simulink model "SIM_4_TANK"  (R2023b)
settings: Solver=VariableStepAuto  StartTime=0.0  StopTime=1200  RelTol=1e-3
values from neighbouring files (symbols this model uses):
  Ts = 3    [NMPC_FOUR_TANKS.m]
  u0 = [55;75]    [NMPC_FOUR_TANKS.m]
libraries: sharedTrackingLibrary x1, mpclib x1, simulink x1
settings Model: Creator=DELL  LastModifiedBy=akeebismail

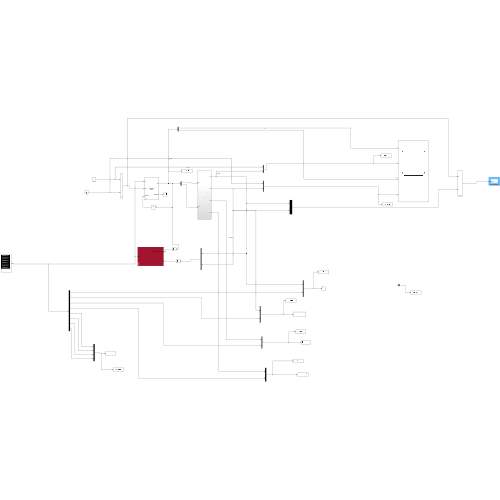
[thumbnail: Simulink's stored preview of the top-level diagram]
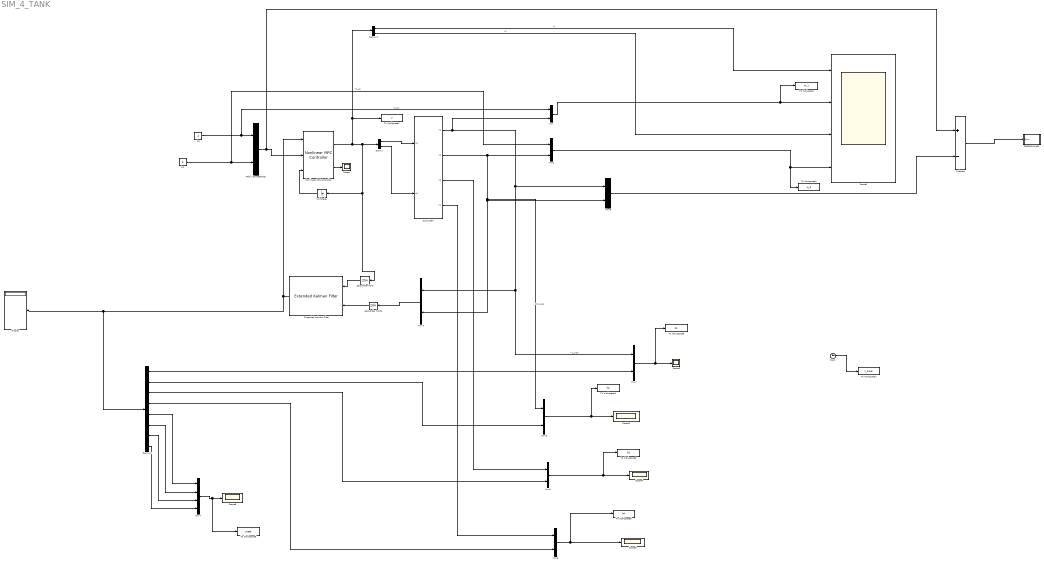
== system SIM_4_TANK ==
  Clock : Clock
  Demux : Demux  Outputs=2
  Demux1 : Demux  Outputs=2
  Demux2 : Demux  Outputs=8
  Display : Display
  Extended Kalman Filter : sharedTrackingLibrary/Extended Kalman Filter  StateTransitionFcn=four_tankStateFcnDT  HasStateTransitionJacobianFcn=off  HasAdditiveProcessNoise=Additive  ProcessNoise=[1e-7;1e-7;1e-7;1e-7;1e-7;1e-7;1e-7;1e-7]  HasTimeVaryingProcessNoise=off  HasStateTransitionFcnExtraArgument=1  InitialState=h0  InitialStateCovariance=[1;1;1;1;1;1;1;1]  MeasurementFcn1=four_tankMeasFcn  HasMeasurementJacobianFcn1=off  HasMeasurementEnablePort1=off  HasAdditiveMeasurementNoise1=Additive  MeasurementNoise1=[1e-2; 1e-2]  HasTimeVaryingMeasurementNoise1=off  HasMeasurementFcnExtraArgument1=0  HasMeasurementWrapping1=off  MeasurementFcn2=myMeasurementFcn  HasMeasurementJacobianFcn2=off  HasMeasurementEnablePort2=off  HasAdditiveMeasurementNoise2=Additive  MeasurementNoise2=1  HasTimeVaryingMeasurementNoise2=off  HasMeasurementFcnExtraArgument2=0  HasMeasurementWrapping2=off  MeasurementFcn3=myMeasurementFcn  HasMeasurementJacobianFcn3=off  HasMeasurementEnablePort3=off  HasAdditiveMeasurementNoise3=Additive  MeasurementNoise3=1  HasTimeVaryingMeasurementNoise3=off  HasMeasurementFcnExtraArgument3=0  HasMeasurementWrapping3=off  MeasurementFcn4=myMeasurementFcn  HasMeasurementJacobianFcn4=off  HasMeasurementEnablePort4=off  HasAdditiveMeasurementNoise4=Additive  MeasurementNoise4=1  HasTimeVaryingMeasurementNoise4=off  HasMeasurementFcnExtraArgument4=0  HasMeasurementWrapping4=off  MeasurementFcn5=myMeasurementFcn  HasMeasurementJacobianFcn5=off  HasMeasurementEnablePort5=off  HasAdditiveMeasurementNoise5=Additive  MeasurementNoise5=1  HasTimeVaryingMeasurementNoise5=off  HasMeasurementFcnExtraArgument5=0  HasMeasurementWrapping5=off  EnableMultirate=off  StateTransitionFcnSampleTime=1  MeasurementFcn1SampleTime=1  MeasurementFcn2SampleTime=1  MeasurementFcn3SampleTime=1  MeasurementFcn4SampleTime=1  MeasurementFcn5SampleTime=1  UseCurrentEstimator=on  OutputStateCovariance=off  DataType=double  SampleTime=Ts  NumberOfMeasurements=1
  Matrix Concatenate : Concatenate  Mode=Multidimensional array  ConcatenateDimension=2
  Mux{,1..6,8} (8 alike) : Mux  Inputs=2
  Mux7 : Mux
  Nonlinear MPC Controller : mpclib/Nonlinear MPC Controller  nlmpcobj=nlobj  UseObjectTs=on  UseMEX=off  md_enabled=off  mvtarget_enabled=off  param_enabled=off  cost_enabled=off  mvseq_enabled=off  stateseq_enabled=off  ovseq_enabled=off  slack_enabled=off  status_enabled=on  ov_min=off  ov_max=off  mv_min=off  mv_max=off  mvrate_min=off  mvrate_max=off  state_min=off  state_max=off  ov_weight=off  mv_weight=off  mvrate_weight=off  ecr_weight=off  nlp_initialize=off
  PERFORMANCE : Subsystem
  Scope{,2..6} (6 alike) : Scope
  Scope1 : Scope  NumInputPorts=4
  Subsystem : Subsystem
  Subtract : Sum  Inputs=+-
  To Workspace : ToWorkspace  VariableName=H_1  SaveFormat=Timeseries  SampleTime=Ts
  To Workspace1 : ToWorkspace  VariableName=H_2  SaveFormat=Timeseries  SampleTime=Ts
  To Workspace2 : ToWorkspace  VariableName=V  SaveFormat=Timeseries  SampleTime=Ts
  To Workspace3 : ToWorkspace  VariableName=h1  SaveFormat=Timeseries  SampleTime=Ts
  To Workspace4 : ToWorkspace  VariableName=h2  SaveFormat=Timeseries  SampleTime=Ts
  To Workspace5 : ToWorkspace  VariableName=h3  SaveFormat=Timeseries  SampleTime=Ts
  To Workspace6 : ToWorkspace  VariableName=h4  SaveFormat=Timeseries  SampleTime=Ts
  To Workspace7 : ToWorkspace  VariableName=t_save  SaveFormat=Timeseries  SampleTime=Ts
  To Workspace8 : ToWorkspace  VariableName=state  SaveFormat=Timeseries  SampleTime=Ts
  Unit Delay : UnitDelay  InitialCondition=u0  SampleTime=-1  HasFrameUpgradeWarning=on
  Zero-Order Hold : ZeroOrderHold  SampleTime=Ts
  Zero-Order Hold1 : ZeroOrderHold  SampleTime=Ts
  h2 : Constant  Value=5
  h3 : Constant  Value=4
  wires:
  h3/1 -> Mux/1, Matrix Concatenate/1  "h1_sp"
  h2/1 -> Matrix Concatenate/2, Mux1/1  "h2_sp"
  Matrix Concatenate/1 -> Subtract/1, Nonlinear MPC Controller/2
  Nonlinear MPC Controller/2 -> Scope/1
  Extended Kalman Filter/1 -> Nonlinear MPC Controller/1, Display/1, Demux2/1
  Nonlinear MPC Controller/1 -> To Workspace2/1, Demux1/1, Zero-Order Hold/1, Unit Delay/1, Demux/1
  Demux/1 -> Subsystem/1(q1)
  Demux/2 -> Subsystem/2(q2)
  Unit Delay/1 -> Nonlinear MPC Controller/3
  Subsystem/1(h1) -> Mux8/1, Mux4/1, Mux2/1, Mux/2  "h1_pred"
  Subsystem/2(h2) -> Mux8/2, Mux4/2, Mux3/1, Mux1/2  "h2_pred"
  Demux1/1 -> Scope1/1  "v1"
  Demux1/2 -> Scope1/3  "v2"
  Mux/1 -> Scope1/2, To Workspace/1
  Mux1/1 -> Scope1/4, To Workspace1/1
  Mux4/1 -> Zero-Order Hold1/1
  Zero-Order Hold1/1 -> Extended Kalman Filter/2
  Zero-Order Hold/1 -> Extended Kalman Filter/1
  Demux2/1 -> Mux2/2
  Demux2/2 -> Mux3/2
  Mux2/1 -> To Workspace3/1, Scope2/1
  Mux3/1 -> To Workspace4/1, Scope3/1
  Demux2/3 -> Mux5/2
  Demux2/4 -> Mux6/2
  Subsystem/3(h3) -> Mux5/1
  Subsystem/4(h4) -> Mux6/1
  Mux5/1 -> To Workspace5/1, Scope4/1
  Mux6/1 -> To Workspace6/1, Scope5/1
  Demux2/5 -> Mux7/1
  Demux2/6 -> Mux7/2
  Demux2/7 -> Mux7/3
  Demux2/8 -> Mux7/4
  Mux7/1 -> To Workspace8/1, Scope6/1
  Clock/1 -> To Workspace7/1
  Mux8/1 -> Subtract/2
  Subtract/1 -> PERFORMANCE/1(Error)

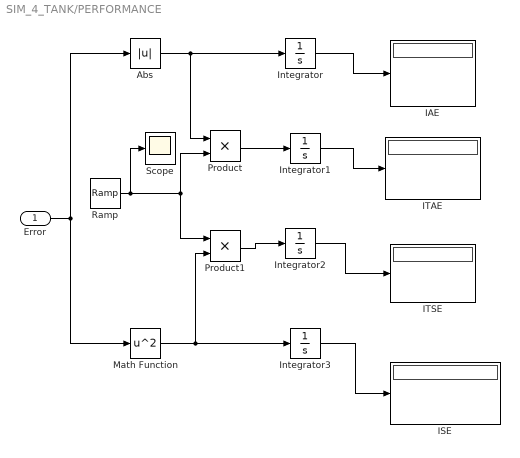
== system SIM_4_TANK/PERFORMANCE ==
  Error : Inport
  Abs : Abs  SaturateOnIntegerOverflow=off
  IAE : Display
  ISE : Display
  ITAE : Display
  ITSE : Display
  Integrator{,1..3} (4 alike) : Integrator
  Math Function : Math  Operator=square  SignedPower=on
  Product : Product  RndMeth=Zero
  Product1 : Product  RndMeth=Zero
  Ramp : simulink/Sources/Ramp  slope=1  start=0  InitialOutput=0
  Scope : Scope
  wires:
  Error/1 -> Math Function/1, Abs/1
  Abs/1 -> Integrator/1, Product/1
  Integrator/1 -> IAE/1
  Ramp/1 -> Product/2, Product1/1, Scope/1
  Math Function/1 -> Integrator3/1, Product1/2
  Product1/1 -> Integrator2/1
  Product/1 -> Integrator1/1
  Integrator3/1 -> ISE/1
  Integrator2/1 -> ITSE/1
  Integrator1/1 -> ITAE/1

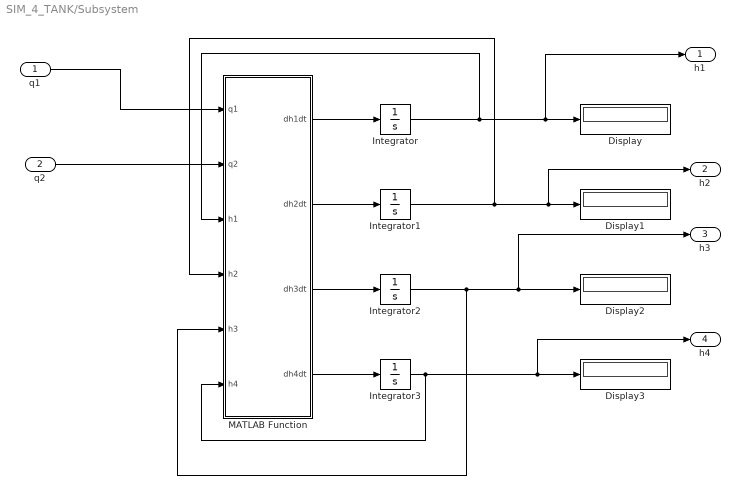
== system SIM_4_TANK/Subsystem ==
  q1 : Inport
  q2 : Inport  Port=2
  Display{,1..3} (4 alike) : Display
  Integrator{,1..3} (4 alike) : Integrator
  MATLAB Function : MATLAB Function  TreatAsAtomicUnit=on
  h1 : Outport
  h2 : Outport  Port=2
  h3 : Outport  Port=3
  h4 : Outport  Port=4
  wires:
  Integrator1/1 -> MATLAB Function/4(h2), h2/1, Display1/1
  q2/1 -> MATLAB Function/2(q2)
  Integrator3/1 -> MATLAB Function/6(h4), h4/1, Display3/1
  q1/1 -> MATLAB Function/1(q1)
  Integrator2/1 -> MATLAB Function/5(h3), h3/1, Display2/1
  MATLAB Function/2(dh2dt) -> Integrator1/1
  MATLAB Function/1(dh1dt) -> Integrator/1
  MATLAB Function/4(dh4dt) -> Integrator3/1
  MATLAB Function/3(dh3dt) -> Integrator2/1
  Integrator/1 -> MATLAB Function/3(h1), h1/1, Display/1

== matlab function SIM_4_TANK/Subsystem/MATLAB Function ==
  data: q1 input; dh1dt output; q2 input; h1 input; h2 input; h3 input; h4 input; dh2dt output; dh3dt output; dh4dt output
function [dh1dt,dh2dt,dh3dt,dh4dt] = fcn(q1,q2,h1,h2,h3,h4)
values = {0.97,0.42,0.74,0.426,0.8542,0.7126,0.7722,0.5149,35,35,39,39,981,0.23,0.19};
[a1,a3,a2,a4,alpha1,alpha3,alpha2,alpha4,A1,A3,A2,A4,g,gamma1,gamma2] = values{:};

%F = k1 * v1;
%F2 = k2 * v2;

    dh1dt = -(a1*alpha1/A1) * sqrt(2 * g * h1) + (a3*alpha3/A1) * sqrt(2 * g * h3) + (gamma1 * q1) / A1;
    dh2dt = -(a2*alpha2/A2) * sqrt(2 * g * h2) + (a4*alpha4/A2) * sqrt(2 * g * h4) + (gamma2 * q2) / A2;
    dh3dt = -(a3*alpha3/A3) * sqrt(2 * g * h3) + ((1 - gamma2) * q2) / A3;
    dh4dt = -(a4*alpha4/A4) * sqrt(2 * g * h4) + ((1 - gamma1) * q1) / A4;

end
